simulink model "gm_encoderN8"  (R2016b)
settings: Solver=FixedStepDiscrete  StartTime=0.0  StopTime=10.0  RelTol=1e-3
settings Model: Creator=hasee  LastModifiedBy=hasee
settings DataIOCC: LimitDataPoints=on  SaveOutput=off  SaveTime=off
settings OptimizationCC: BlockReduction=off  ConditionallyExecuteInputs=off  DefaultParameterBehavior=Inlined  LifeSpan=inf
settings DebuggingCC: AlgebraicLoopMsg=error  InheritedTsInSrcMsg=none  SingleTaskRateTransMsg=error  AllowSymbolicDim=off  StrictBusMsg=ErrorOnBusTreatedAsVector  SFUnexpectedBacktrackingDiag=warning  SFNoUnconditionalDefaultTransitionDiag=warning  SFExecutionAtInitializationDiag=none
settings HardwareCC: ProdBitPerPointer=32  ProdBitPerSizeT=32  ProdBitPerPtrDiffT=32  ProdLargestAtomicFloat=None  ProdIntDivRoundTo=Undefined  ProdEndianess=Unspecified  ProdWordSize=32  ProdHWDeviceType=ASIC/FPGA->ASIC/FPGA  ProdEqTarget=off
settings GRTTargetCC: TargetLangStandard=C89/C90 (ANSI)  GeneratePreprocessorConditionals=Disable all
settings ConfigComp: CovScope=ReferencedModels  CovMetricSettings=dw  CovHtmlReporting=on  CovSaveCumulativeToWorkspaceVar=on  CovSaveSingleToWorkspaceVar=on  CovExternalEMLEnable=off  CovSFcnEnable=off

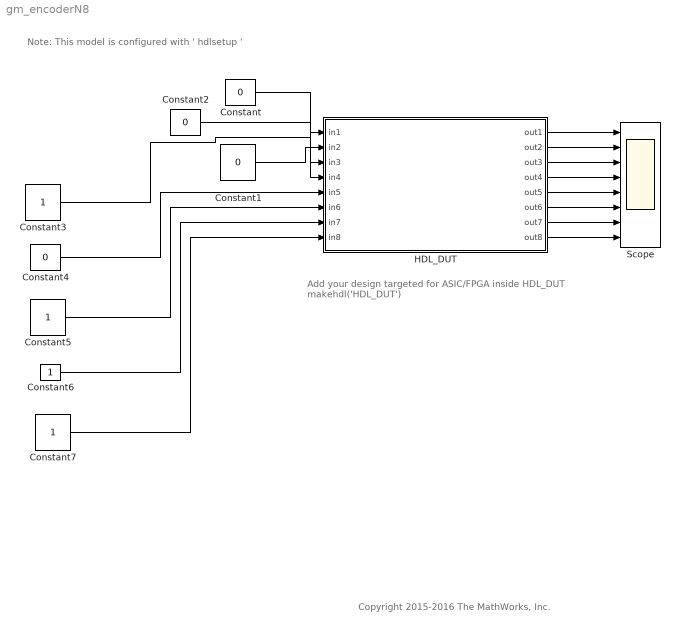
== system gm_encoderN8 ==
  note: Copyright 2015-2016 The MathWorks, Inc.
  note: Add your design targeted for ASIC/FPGA inside HDL_DUT
      | makehdl('HDL_DUT')
  note: Note: This model is configured with ' hdlsetup '
  Constant{,1..2,4} (4 alike) : Constant  Value=0  OutDataTypeStr=boolean  SampleTime=-1
  Constant{3,5..7} (4 alike) : Constant  OutDataTypeStr=boolean  SampleTime=-1
  HDL_DUT : Subsystem
  Scope : Scope  NumInputPorts=8
  wires:
  Constant7/1 -> HDL_DUT/8(in8)
  Constant6/1 -> HDL_DUT/7(in7)
  Constant5/1 -> HDL_DUT/6(in6)
  Constant4/1 -> HDL_DUT/5(in5)
  Constant3/1 -> HDL_DUT/4(in4)
  Constant2/1 -> HDL_DUT/3(in3)
  HDL_DUT/8(out8) -> Scope/8
  HDL_DUT/7(out7) -> Scope/7
  HDL_DUT/6(out6) -> Scope/6
  HDL_DUT/5(out5) -> Scope/5
  HDL_DUT/4(out4) -> Scope/4
  HDL_DUT/3(out3) -> Scope/3
  HDL_DUT/2(out2) -> Scope/2
  HDL_DUT/1(out1) -> Scope/1
  Constant1/1 -> HDL_DUT/2(in2)
  Constant/1 -> HDL_DUT/1(in1)

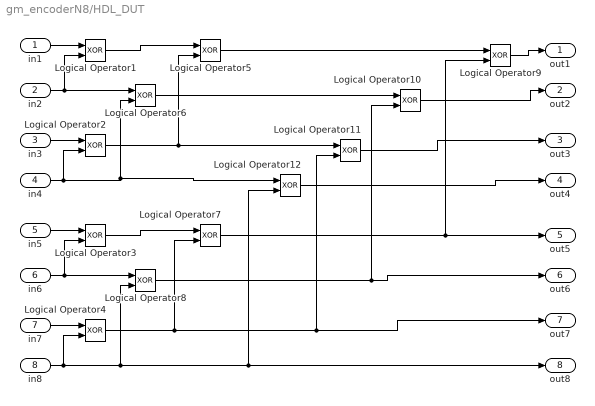
== system gm_encoderN8/HDL_DUT ==
  in1 : Inport
  in2 : Inport  Port=2
  in3 : Inport  Port=3
  in4 : Inport  Port=4
  in5 : Inport  Port=5
  in6 : Inport  Port=6
  in7 : Inport  Port=7
  in8 : Inport  Port=8
  Logical Operator{1..12} (12 alike) : Logic  Operator=XOR  AllPortsSameDT=off  OutDataTypeStr=boolean
  out1 : Outport
  out2 : Outport  Port=2
  out3 : Outport  Port=3
  out4 : Outport  Port=4
  out5 : Outport  Port=5
  out6 : Outport  Port=6
  out7 : Outport  Port=7
  out8 : Outport  Port=8
  wires:
  Logical Operator12/1 -> out4/1
  Logical Operator11/1 -> out3/1
  Logical Operator8/1 -> out6/1, Logical Operator10/2
  Logical Operator10/1 -> out2/1
  Logical Operator6/1 -> Logical Operator10/1
  Logical Operator4/1 -> Logical Operator11/2, out7/1, Logical Operator7/2
  Logical Operator3/1 -> Logical Operator7/1
  in7/1 -> Logical Operator4/1
  in8/1 -> Logical Operator12/2, out8/1, Logical Operator8/2, Logical Operator4/2
  in6/1 -> Logical Operator3/2, Logical Operator8/1
  in5/1 -> Logical Operator3/1
  Logical Operator7/1 -> out5/1, Logical Operator9/2
  Logical Operator9/1 -> out1/1
  Logical Operator5/1 -> Logical Operator9/1
  Logical Operator2/1 -> Logical Operator5/2, Logical Operator11/1
  Logical Operator1/1 -> Logical Operator5/1
  in3/1 -> Logical Operator2/1
  in4/1 -> Logical Operator6/2, Logical Operator12/1, Logical Operator2/2
  in2/1 -> Logical Operator1/2, Logical Operator6/1
  in1/1 -> Logical Operator1/1
